simulink model "MPPT"  (R2014a)
settings: Solver=ode45  StartTime=0.0  StopTime=10.0  RelTol=1e-3
values from neighbouring files (symbols this model uses):
  Array_Voc = [0.328644000009 2.76811 3.09396940822 3.26133568944 3.36629977409 3.44398192097 3.50365713438 3.55225637345 3.59363766529 3.63021764721 3.6624 3.69037314882 ... (101 elements, 101x1)]    [Array_Voc.mat]
  ArrayCurrent = [1.05303e-05 0.0329007487024 0.0659314357778 0.100205 0.132978217474 0.166891516648 0.200872978445 0.234107600227 0.267513340222 0.302009988541 0.336322 0.36979130469 ... (44440 elements, 101x440)]    [ArrayCurrent.mat]    (also in Genrate_SC_mod.m = fitresult_normal_g42(V,G); temp3.m = fitresult(V,G))
  ArrayVoltage = [0 0.01 0.02 0.03 0.04 0.05 0.06 0.07 0.08 0.09 0.1 0.11 ... (440 elements, 1x440)]    [ArrayVoltage.mat]    (also in Genrate_SC_mod.m = (0:0.01:max(Voltage)); temp3.m = (0:0.01:max(Voltage)))
  Irradiance = (min(Lux):50:max(Lux))    [Genrate_SC_mod.m]    (also in Irradiance.mat = [0 50 100 150 200 250 300 350 400 450 500 550 ... (101 eleme; temp3.m)
libraries: powerlib x5, simulink_extras x1
settings Model: Creator=kartik.karuna  LastModifiedBy=kartik.karuna

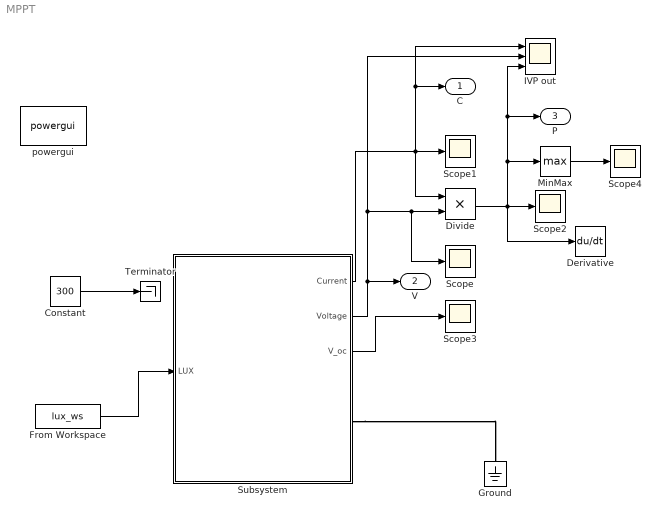
== system MPPT ==
  Constant : Constant  Value=300
  Derivative : Derivative
  Divide : Product  Inputs=**
  From Workspace : FromWorkspace  VariableName=lux_ws  OutDataTypeStr=double  SampleTime=0
  Ground : powerlib/Elements/Ground  LConnTagsString=a
  IVP out : Scope  NumInputPorts=3
      settings: YMin=-5~-5~-5  YMax=5~5~5  SaveName=Simulation_out
  MinMax : MinMax  Function=max
  Scope{,1..4} (5 alike) : Scope
      Scope2 settings: SaveName=ScopeData2
      Scope3 settings: SaveName=ScopeData3
      Scope4 settings: SaveName=ScopeData4
  Subsystem : Subsystem
  Terminator : Terminator
  powergui : powerlib/powergui  Priority=1  SimulationMode=Continuous  SolverType=Tustin  SampleTime=50e-6  frequency=50  SPID=off  DisableSnubberDevices=off  DisableRonSwitches=off  DisableVfSwitches=off  SwTol=0  Interpol=off  DisplayEquations=off  Ts=0  methode=off  frequencyindice=0  Pbase=100e6  ErrMax=1e-4  Iterations=50  UnitsV=kV  UnitsW=MW  FunctionMessages=off  echomessages=off  HookPort=off  EnableUseOfTLC=off  x0status=blocks  RestoreLinks=warning  ResistiveCurrentMeasurement=off  Frange=[0:2:500]  Ylog=off  Xlog=on  ShowGrid=off  save=off  variable=ZData  structure=0  ZoomFFT=off  StartTime=0.0  cycles=1  DisplayStyle=1  fundamental=60  FreqAxis=off  MaxFrequency=1000  frequencyindicesteady=1  RmsSteady=1  display=off
  "C " : Outport  InitialOutput=0
  V : Outport  Port=2  InitialOutput=0
  P : Outport  Port=3  InitialOutput=0
  wires:
  Subsystem/1(Current) -> IVP out/1, "C "/1, Divide/1, Scope1/1
  Subsystem/2(Voltage) -> IVP out/2, Scope/1, Divide/2, V/1
  Subsystem/3("V_oc ") -> Scope3/1
  Divide/1 -> Derivative/1, MinMax/1, IVP out/3, P/1, Scope2/1
  MinMax/1 -> Scope4/1
  Constant/1 -> Terminator/1
  From Workspace/1 -> Subsystem/1(LUX)
  connections:
  Subsystem/RConn2 -- Ground/LConn1

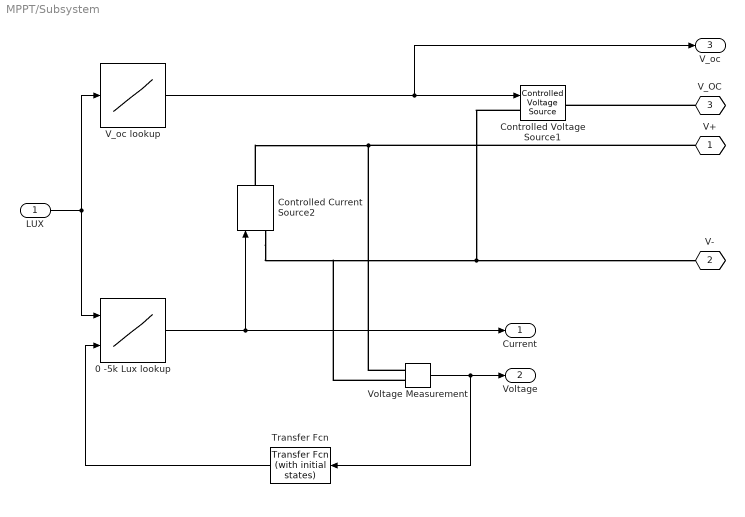
== system MPPT/Subsystem ==
  LUX : Inport
  0 -5k Lux lookup : Lookup_n-D  BreakpointsForDimension1=Irradiance  BreakpointsForDimension2=ArrayVoltage  Table=ArrayCurrent  RndMeth=Simplest  InputSameDT=on
  Controlled Current Source2 : powerlib/Electrical Sources/Controlled Current Source  Initialize=on  Source_Type=DC  Amplitude=0  Phase=0  Frequency=0  Measurements=None
  Controlled Voltage Source1 : powerlib/Electrical Sources/Controlled Voltage Source  Initialize=on  Source_Type=AC  Amplitude=0  Phase=0  Frequency=0  Measurements=Voltage
  Transfer Fcn : simulink_extras/Additional Linear/Transfer Fcn (with initial states)  N=[1]  D="[.0001  1]"  X0=0
  V_oc lookup : Lookup_n-D  NumberOfTableDimensions=1  BreakpointsForDimension1=Irradiance  Table=Array_Voc  RndMeth=Simplest  InputSameDT=on
  Voltage Measurement : powerlib/Measurements/Voltage Measurement  PhasorSimulation=off  OutputType=Complex  PSBequivalent=0
  V+ : PMIOPort  Tag=PMCPort  Port=1  Side=Right
  V- : PMIOPort  Tag=PMCPort  Port=2  Side=Right
  V_OC : PMIOPort  Tag=PMCPort  Port=3  Side=Right
  Current : Outport
  Voltage : Outport  Port=2
  "V_oc " : Outport  Port=3
  wires:
  LUX/1 -> 0 -5k Lux lookup/1, V_oc lookup/1
  Voltage Measurement/1 -> Voltage/1, Transfer Fcn/1
  Transfer Fcn/1 -> 0 -5k Lux lookup/2
  0 -5k Lux lookup/1 -> Controlled Current Source2/1, Current/1
  V_oc lookup/1 -> "V_oc "/1, Controlled Voltage Source1/1
  connections:
  Controlled Current Source2/RConn1 -- V+/RConn1 -- Voltage Measurement/LConn1
  Controlled Voltage Source1/LConn1 -- Voltage Measurement/LConn2 -- Controlled Current Source2/LConn1 -- V-/RConn1
  V_OC/RConn1 -- Controlled Voltage Source1/RConn1
